simulink model "LIST3_INTEGRADOR_sim_new"  (R2024a)
settings: Solver=VariableStepAuto  StartTime=0.0  StopTime=10.0  RelTol=1e-3
values from neighbouring files (symbols this model uses):
  C = [1 3]    [LIST3_Q2.m]    (also in LIST3_Q5_a.m = SS2_z.C; LIST3_Q5_b.m = SS2_z.C; LIST3_Q6_a.m = [1 0]; LIST3_Q6_b.m = [1 0])
  G = [0.6 0;         0 0.4]    [LIST3_Q2.m]    (also in LIST3_Q4.m = [1 1;      0 1]; LIST3_Q5_a.m = SS2_z.A; LIST3_Q5_b.m = SS2_z.A; LIST3_Q6_a.m = [0.8815 0.4562;      -0.4562 0.7903])
  H = [1;         5]    [LIST3_Q2.m]    (also in LIST3_Q4.m = [0.5;       1]; LIST3_Q5_a.m = SS2_z.B; LIST3_Q5_b.m = SS2_z.B; LIST3_Q6_a.m = [0.1185;      0.4562])
  K = [k1 k2]    [LIST3_Q4.m]    (also in LIST3_Q5_b.m = K(1:end-1); LIST3_Q6_b.m = K(1:end-1))
  Ki = K(end)    [LIST3_Q5_b.m]    (also in LIST3_Q6_b.m)
  Ts = 0.01    [LIST3_Q5_a.m]    (also in LIST3_Q5_b.m; LIST3_Q6_a.m = 1; LIST3_Q6_b.m = 1; LIST3_Q6_c.m = 1)
settings Model: Creator=ribei  LastModifiedBy=brend
settings SolverCC: AlgebraicLoopSolver=TrustRegion
settings DebuggingCC: ArithmeticOperatorsInVariantConditions=warning
settings SFSimCC: CustomCodeUndefinedFunction=UseInterfaceOnly
settings RTWCC: GPUComputeCapability=3.5
settings CodeAppCC: StateflowObjectComments=on

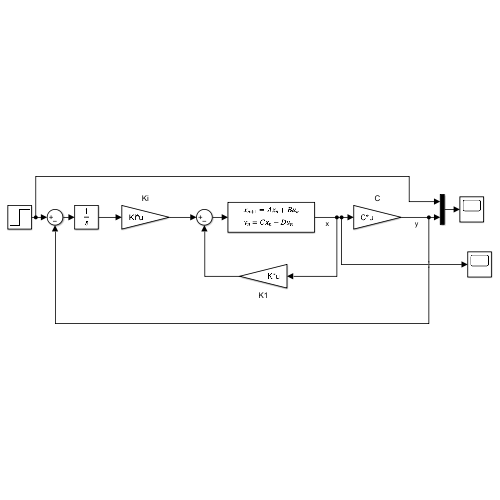
[thumbnail: Simulink's stored preview of the top-level diagram]
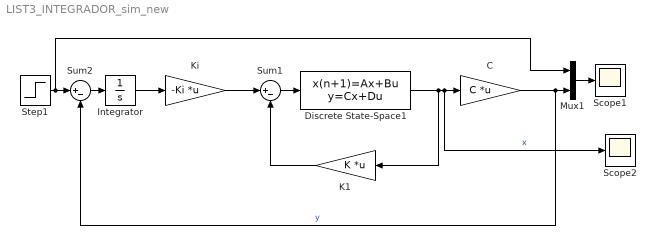
== system LIST3_INTEGRADOR_sim_new ==
  C : Gain  Gain=C  Multiplication=Matrix(K*u)
  Discrete State-Space1 : DiscreteStateSpace  A=G  B=H  C=eye(2)  D=zeros(2,1)  InitialCondition=[0; 0]  SampleTime=Ts
  Integrator : Integrator
  K1 : Gain  Gain=K  Multiplication=Matrix(K*u)
  Ki : Gain  Gain=-Ki  Multiplication=Matrix(K*u)
  Mux1 : Mux  Inputs=2
  Scope1 : Scope
  Scope2 : Scope
  Step1 : Step  SampleTime=0
  Sum1 : Sum  Inputs=|+-
  Sum2 : Sum  Inputs=|+-
  wires:
  Mux1/1 -> Scope1/1
  Step1/1 -> Mux1/1, Sum2/1
  Sum1/1 -> Discrete State-Space1/1
  Discrete State-Space1/1 -> Scope2/1, C/1, K1/1  "x"
  K1/1 -> Sum1/2
  Ki/1 -> Sum1/1
  C/1 -> Sum2/2, Mux1/2  "y"
  Sum2/1 -> Integrator/1
  Integrator/1 -> Ki/1
